simulink model "Trim_Model"  (R2012b)
settings: Solver=ode23tb  StartTime=0.0  StopTime=inf  FixedStep=0.001  MaxStep=0.01  RelTol=1e-5
values from neighbouring files (symbols this model uses):
  a = 2.1117    [SetupComplete.m]
  A_x = 0.015    [SetupComplete.m]
  A_y = A_x    (= 0.015)    [SetupComplete.m]
  A_z = 0.16    [SetupComplete.m]
  C_d0 = 0.00209    [SetupComplete.m]
  C_x = 1.2    [SetupComplete.m]
  C_y = C_x    (= 1.2)    [SetupComplete.m]
  C_z = 2.2    [SetupComplete.m]
  CG_0 = [0,0,0.02]'    [SetupComplete.m]
  h = 0.08    [SetupComplete.m]
  h_FA = 0.02    [SetupComplete.m]
  h_M = 0.064    [SetupComplete.m]
  I_BAC_0 = [ Ix,0,Ixz;0,Iy,0;Ixz,0,Iz]    [SetupComplete.m]
  I_prop = 1/4*M_eq*R^2*diag([1,1,2])    [SetupComplete.m]
  I_tube = [1/2*M_tube*R_tube_eq^2,0,  0  ;           0 ,1/3*M_tube*l_arm^2,0;             0  ,0,1/3*M_tube*l_arm^2]    [SetupComplete.m]
  Initial_Omegas = [1;1;1]*Omega_hover    [Run3Copter.m]
  Initial_Torques = [1;1;1]*Torque_hover    [Run3Copter.m]
  J_FA = I_prop(1,1) + m_prop*h^2  + m_FA*h_FA^2 + m_M*h_M^2    [SetupComplete.m]
  J_T = J_m+1/2*M_eq*R^2    (= 2.000642e-05)    [SetupComplete.m]
  l = 0.345    [SetupComplete.m]
  l_arm = 0.264    [SetupComplete.m]
  m = 3.51    [SetupComplete.m]
  m_0 = 2.61    [SetupComplete.m]
  m_FA = 0.02    [SetupComplete.m]
  m_M = 0.300    (= 0.3)    [SetupComplete.m]
  m_prop = 0.02    [SetupComplete.m]
  Omega_hover = 570    [SetupComplete.m]
  R = 0.1778    [SetupComplete.m]
  rho = 1.15    [SetupComplete.m]
  Rotation_sign = [ 1,-1,-1]    [SetupComplete.m]
  sigma = b*c/(pi*R)    (= 0.107416159567)    [SetupComplete.m]
  Tau_motors = 0.06    [SetupComplete.m]
  theta_0 = 0.38397    [SetupComplete.m]
  theta_1 = -0.2967    [SetupComplete.m]
  Throttle_Hover = X(1)/16    [SetupComplete.m]
  v_i0 = sqrt( 1/3*m*g/(2*rho*pi*R^2)  )    [SetupComplete.m]
undefined symbols (not defined in the file or in its folder): Omega_TTO, Throtle_TTO, Torque_TTO, v_i_adim, Vx_adim, Vz_adim
libraries: vrlib x15, dspmtrx3 x11, simulink_extras x4, aerolibtransform2 x1
(part 1 of 2)
settings Model: ExtModeTrigDuration=5000  Creator=DavidTorres  LastModifiedBy=David
settings SolverCC: SolverResetMethod=Robust  PositivePriorityOrder=on
settings DataIOCC: ExternalInput=getinputstruct(op_trim1)  InitialState=getstatestruct(op_trim1)  SignalLoggingSaveFormat=ModelDataLogs  Refine=10
settings OptimizationCC: InlineParams=on
settings DebuggingCC: FcnCallInpInsideContextMsg=UseLocalSettings
settings RTWCC: SystemTargetFile=quarc_windows.tlc  TemplateMakefile=quarc_default_tmf  Description=QUARC Win32 Target  ProcessScript=quarc_windows_make_rtw_hook
settings STFCustomTargetCC: TargetPreCompLibLocation=C:\PROGRA~2\QUARC\lib\2011a\windows\release  CodeReplacementLibrary=ANSI_C  GeneratePreprocessorConditionals=Disable all  SystemTargetFile=quarc_windows.tlc
settings GRTTargetCC: TargetPreCompLibLocation=C:\PROGRA~2\QUARC\lib\2011a\windows\release  ParMdlRefBuildCompliant=off  CompOptLevelCompliant=off  ConcurrentExecutionCompliant=off  CombineOutputUpdateFcns=off  MatFileLogging=off  GRTInterface=on  ExtMode=on  ExtModeMexFile=quarc_comm

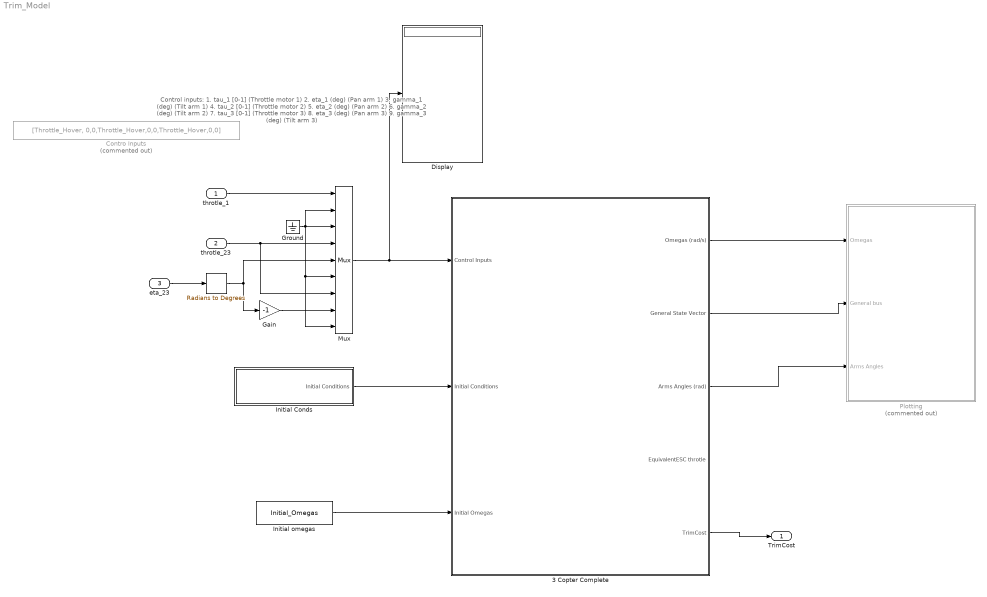
== system Trim_Model ==
  note: Control inputs:
      | 1. tau_1 [0-1] (Throttle motor 1)
      | 2. eta_1 (deg)  (Pan arm 1)
      | 3. gamma_1 (deg)  (Tilt arm 1)
      |
      | 4. tau_2 [0-1] (Throttle motor 2)
      | 5. eta_2 (deg)  (Pan arm 2)
      | 6. gamma_2 (deg)  (Tilt arm 2)
      |
      | 7. tau_3 [0-1] (Throttle motor 3)
      | 8. eta_3 (deg)  (Pan arm  3)
      | 9. gamma_3 (deg)  (Tilt arm 3)
  throtle_1 : Inport
  throtle_23 : Inport  Port=2
  eta_23 : Inport  Port=3
  " " : simulink_extras/Transformations/Radians to Degrees
  3 Copter Complete : Subsystem  TreatAsAtomicUnit=on
  Contro Inputs : Constant  Commented=on  Value=[Throttle_Hover, 0,0,Throttle_Hover,0,0,Throttle_Hover,0,0]
  Display : Display
  Gain : Gain  Gain=-1
  Ground : Ground
  Initial Conds : Subsystem  TreatAsAtomicUnit=on
  Initial omegas : Constant  Value=Initial_Omegas
  Mux : Mux  Inputs=9
  Plotting : Subsystem  Commented=on
  TrimCost : Outport
  wires:
  Initial omegas/1 -> 3 Copter Complete/3(Initial Omegas)
  Initial Conds/1(Initial Conditions) -> 3 Copter Complete/2(Initial Conditions)
  Mux/1 -> Display/1, 3 Copter Complete/1(Control Inputs)
  3 Copter Complete/2(General State Vector) -> Plotting/2(General bus)
  3 Copter Complete/1(Omegas (rad/s)) -> Plotting/1(Omegas)
  3 Copter Complete/3(Arms Angles (rad)) -> Plotting/3(Arms Angles)
  3 Copter Complete/5(TrimCost) -> TrimCost/1
  throtle_1/1 -> Mux/1
  throtle_23/1 -> Mux/7, Mux/4
  Ground/1 -> Mux/2, Mux/6, Mux/9, Mux/3
  eta_23/1 -> " "/1
  " "/1 -> Gain/1, Mux/5
  Gain/1 -> Mux/8

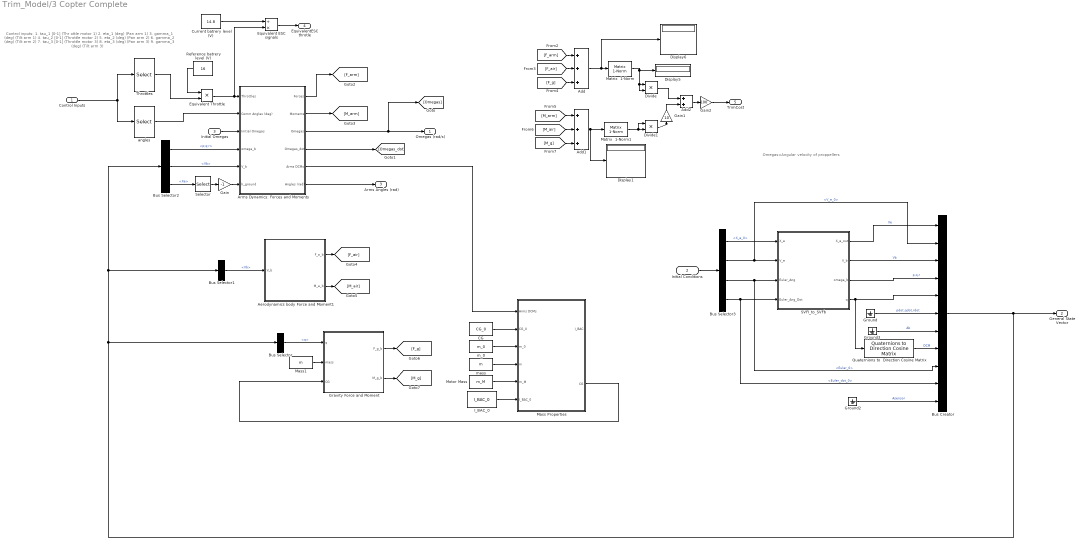
== system Trim_Model/3 Copter Complete ==
  note: Omegas=Angular velocity of proppellers
  note: Control inputs:
      | 1. tau_1 [0-1] (Thr ottle motor 1)
      | 2. eta_1 (deg)  (Pan arm 1)
      | 3. gamma_1 (deg)  (Tilt arm 1)
      |
      | 4. tau_2 [0-1] (Throttle motor 2)
      | 5. eta_2 (deg)  (Pan arm 2)
      | 6. gamma_2 (deg)  (Tilt arm 2)
      |
      | 7. tau_3 [0-1] (Throttle motor 3)
      | 8. eta_3 (deg)  (Pan arm  3)
      | 9. gamma_3 (deg)  (Tilt arm 3)
  Control Inputs : Inport
  Initial Conditions : Inport  Port=2
  Initial Omegas : Inport  Port=3
  Add : Sum  Inputs=+++
  Add1 : Sum  Inputs=+++
  Add2 : Sum
  Aerodynamics body Force and Moment1 : MATLAB Function  TreatAsAtomicUnit=on
  Arms Dynamics: Forces and Moments : Subsystem  TreatAsAtomicUnit=on
  Bus Creator : BusCreator  Inputs=11
  Bus Selector : BusSelector  OutputSignals=q
  Bus Selector1 : BusSelector  OutputSignals=Vb
  Bus Selector2 : BusSelector  OutputSignals=p;q;r,Vb,Xe
  Bus Selector3 : BusSelector  OutputSignals=X_e_0,V_e_0,Euler_0,Euler_dot_0
  CG : Constant  Value=CG_0
  Current batrery level (V) : Constant  Value=14.8
  Display1 : Display
  Display5 : Display
  Display6 : Display
  Divide : Product  Inputs=**
  Divide1 : Product  Inputs=**
  Equivalent ESC signals : Product  Inputs=/*
  Equivalent Throttle : Product  Inputs=**
  Gain : Gain  Gain=-1
  Gain1 : Gain  Gain=10
  Gain2 : Gain  Gain=100
  Gravity Force and Moment : MATLAB Function  TreatAsAtomicUnit=on
  Ground : Ground
  Ground2 : Ground
  Ground3 : Ground
  I_BAC_0 : Constant  Value=I_BAC_0
  Mass Properties : Subsystem  TreatAsAtomicUnit=on
  Mass1 : Constant  Value=m
  Matrix  1-Norm : dspmtrx3/Matrix  1-Norm  outputDataTypeStr=Inherit: Same as accumulator  outputLastDataTypeStr=Inherit: Same as accumulator  outputMin=[]  outputMax=[]  roundingMode=Floor  overflowMode=off
  Matrix  1-Norm1 : dspmtrx3/Matrix  1-Norm  outputDataTypeStr=Inherit: Same as accumulator  outputLastDataTypeStr=Inherit: Same as accumulator  outputMin=[]  outputMax=[]  roundingMode=Floor  overflowMode=off
  Motor Mass : Constant  Value=m_M
  Quaternions to  Direction Cosine Matrix : aerolibtransform2/Quaternions to  Direction Cosine Matrix
  Reference batrery level (V) : Constant  Value=16
  SVFI_to_SVFb : MATLAB Function  TreatAsAtomicUnit=on
  Selector : Selector  InputPortWidth=3  IndexOptions=Index vector (dialog)  Indices=3  OutputSizes=1
  Throttles : Selector  InputPortWidth=9  IndexOptions=Index vector (dialog)  Indices=[1,4,7]  OutputSizes=1
  "angles " : Selector  InputPortWidth=9  IndexOptions=Index vector (dialog)  Indices=[2,3,5,6,8,9]  OutputSizes=1
  m_0 : Constant  Value=m_0
  mass : Constant  Value=m
  Omegas (rad/s) : Outport
  General State Vector : Outport  Port=2
  Arms Angles (rad) : Outport  Port=3
  EquivalentESC throtle : Outport  Port=4
  TrimCost : Outport  Port=5
  wires:
  SVFI_to_SVFb/3(omega_b) -> Bus Creator/4  "p,q,r"
  SVFI_to_SVFb/2(V_b) -> Bus Creator/3  "Vb"
  SVFI_to_SVFb/4(q) -> Quaternions to  Direction Cosine Matrix/1, Bus Creator/5
  Ground/1 -> Bus Creator/6  "pdot,qdot,rdot"
  SVFI_to_SVFb/1(X_e_out) -> Bus Creator/1  "Xe"
  Ground3/1 -> Bus Creator/7  "Ab"
  Bus Selector/1 -> Gravity Force and Moment/1(q)  "<q>"
  Bus Selector1/1 -> Aerodynamics body Force and Moment1/1(V_b)  "<Vb>"
  Bus Selector2/1 -> Arms Dynamics: Forces and Moments/4(omega_b)  "<p;q;r>"
  Bus Selector2/2 -> Arms Dynamics: Forces and Moments/5(V_b)  "<Vb>"
  Mass1/1 -> Gravity Force and Moment/2(mass)
  Mass Properties/2(CG) -> Gravity Force and Moment/3(CG)
  Arms Dynamics: Forces and Moments/4(Omegas_dot) -> [Omegas_dot]
  Initial Omegas/1 -> Arms Dynamics: Forces and Moments/3(Initial Omegas)
  Bus Selector2/3 -> Selector/1  "<Xe>"
  Selector/1 -> Gain/1
  Gain/1 -> Arms Dynamics: Forces and Moments/6(h_ground)
  Arms Dynamics: Forces and Moments/1(Forces) -> [F_arm]
  Arms Dynamics: Forces and Moments/2(Moments) -> [M_arm]
  Aerodynamics body Force and Moment1/1(F_a_b) -> [F_air]
  Aerodynamics body Force and Moment1/2(M_a_b) -> [M_air]
  Gravity Force and Moment/1(F_g_b) -> [F_g]
  Gravity Force and Moment/2(M_g_b) -> [M_g]
  [F_arm] -> Add/1
  [F_air] -> Add/2
  [F_g] -> Add/3
  [M_arm] -> Add1/1
  [M_g] -> Add1/3
  [M_air] -> Add1/2
  Ground2/1 -> Bus Creator/11  "Asensor"
  Throttles/1 -> Equivalent Throttle/2
  Control Inputs/1 -> "angles "/1, Throttles/1
  "angles "/1 -> Arms Dynamics: Forces and Moments/2(Comm Angles (deg))
  Arms Dynamics: Forces and Moments/5(Arms DCMs) -> Mass Properties/1(Arms DCMs)
  CG/1 -> Mass Properties/2(CG_0)
  Motor Mass/1 -> Mass Properties/5(m_M)
  I_BAC_0/1 -> Mass Properties/6(I_BAC_0)
  m_0/1 -> Mass Properties/3(m_0)
  mass/1 -> Mass Properties/4(m)
  Arms Dynamics: Forces and Moments/3(Omegas) -> [Omegas], Omegas (rad/s)/1
  Arms Dynamics: Forces and Moments/6(Angles (rad)) -> Arms Angles (rad)/1
  Bus Creator/1 -> Bus Selector2/1, Bus Selector1/1, Bus Selector/1, General State Vector/1
  Equivalent Throttle/1 -> Equivalent ESC signals/2, Arms Dynamics: Forces and Moments/1(Throttles)
  Reference batrery level (V)/1 -> Equivalent Throttle/1
  Current batrery level (V)/1 -> Equivalent ESC signals/1
  Equivalent ESC signals/1 -> EquivalentESC throtle/1
  Initial Conditions/1 -> Bus Selector3/1
  Bus Selector3/1 -> SVFI_to_SVFb/1(X_e)  "<X_e_0>"
  Bus Selector3/2 -> Bus Creator/2, SVFI_to_SVFb/2(V_e)  "<V_e_0>"
  Bus Selector3/3 -> Bus Creator/9, SVFI_to_SVFb/3(Euler_Ang)  "<Euler_0>"
  Bus Selector3/4 -> Bus Creator/10, SVFI_to_SVFb/4(Euler_Ang_Dot)  "<Euler_dot_0>"
  Quaternions to  Direction Cosine Matrix/1 -> Bus Creator/8  "DCM"
  Add/1 -> Display6/1, Matrix  1-Norm/1
  Add1/1 -> Display1/1, Matrix  1-Norm1/1
  Add2/1 -> Gain2/1
  Gain1/1 -> Add2/2
  Matrix  1-Norm1/1 -> Divide1/1, Divide1/2
  Matrix  1-Norm/1 -> Divide/2, Divide/1, Display5/1
  Gain2/1 -> TrimCost/1
  Divide/1 -> Add2/1
  Divide1/1 -> Gain1/1

== system Trim_Model/Initial Conds ==
  Bus Creator : BusCreator
  Ini Position X_e_0 : Constant  Value=[0;0;-20]
  Initial Attitude Euler_0 : Constant  Value=[deg2rad(0);deg2rad(0);deg2rad(0)]
  Initial Attitude Rate  Euler_dot_0 : Constant  Value=[deg2rad(0);deg2rad(0);deg2rad(0)]
  Initial Velocity V_e_0 : Constant  Value=[0;0;0]
  Initial Conditions : Outport
  wires:
  Ini Position X_e_0/1 -> Bus Creator/1  "X_e_0"
  Initial Velocity V_e_0/1 -> Bus Creator/2  "V_e_0"
  Initial Attitude Euler_0/1 -> Bus Creator/3  "Euler_0"
  Initial Attitude Rate  Euler_dot_0/1 -> Bus Creator/4  "Euler_dot_0"
  Bus Creator/1 -> Initial Conditions/1

== system Trim_Model/Plotting ==
  Omegas : Inport
  General bus : Inport  Port=2
  Arms Angles : Inport  Port=3
  Bus Selector : BusSelector  OutputSignals=euler,Xe
  Bus Selector1 : BusSelector  OutputSignals=Angles Arm 1,Angles Arm 2,Angles Arm 3
  Scope : Scope  NumInputPorts=2
      settings: YMin=-3.5~-110  YMax=3.5~40
  Scope1 : Scope
      settings: TimeRange=5  YMin=0  YMax=700
  Scope2 : Scope  NumInputPorts=3
      settings: ShowLegends=on  YMin=-5~-5~-5  YMax=5~5~5  SaveName=ScopeData2
  wires:
  General bus/1 -> Bus Selector/1
  Bus Selector/1 -> Scope/1  "<euler>"
  Omegas/1 -> Scope1/1  "Omegas"
  Arms Angles/1 -> Bus Selector1/1
  Bus Selector1/3 -> Scope2/3  "<Angles Arm 3>"
  Bus Selector1/2 -> Scope2/2  "<Angles Arm 2>"
  Bus Selector1/1 -> Scope2/1  "<Angles Arm 1>"
  Bus Selector/2 -> Scope/2  "<Xe>"

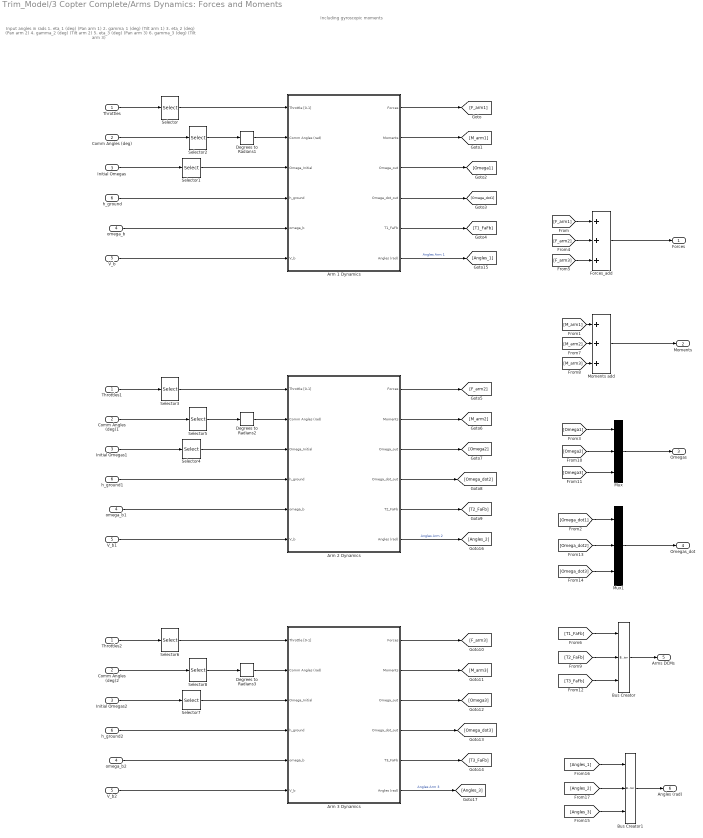
== system Trim_Model/3 Copter Complete/Arms Dynamics: Forces and Moments ==
  note: Including gyroscopic moments
  note: Input angles in rads
      |
      | 1. eta_1 (deg)  (Pan arm 1)
      | 2. gamma_1 (deg)  (Tilt arm 1)
      |
      | 3. eta_2 (deg)  (Pan arm 2)
      | 4. gamma_2 (deg)  (Tilt arm 2)
      |
      | 5. eta_3 (deg)  (Pan arm  3)
      | 6. gamma_3 (deg)  (Tilt arm 3)
  Throttles : Inport
  Comm Angles (deg) : Inport  Port=2
  Initial Omegas : Inport  Port=3
  omega_b : Inport  Port=4
  V_b : Inport  Port=5
  h_ground : Inport  Port=6
  Arm 1 Dynamics : Subsystem  TreatAsAtomicUnit=on
  Arm 2 Dynamics : Subsystem  TreatAsAtomicUnit=on
  Arm 3 Dynamics : Subsystem  TreatAsAtomicUnit=on
  Bus Creator : BusCreator  Inputs=3
  Bus Creator1 : BusCreator  Inputs=3
  Comm Angles (deg)1 : InportShadow  Port=2
  Comm Angles (deg)2 : InportShadow  Port=2
  Degrees to Radians1 : simulink_extras/Transformations/Degrees to Radians
  Degrees to Radians2 : simulink_extras/Transformations/Degrees to Radians
  Degrees to Radians3 : simulink_extras/Transformations/Degrees to Radians
  Forces_add : Sum  Inputs=+++
  Initial Omegas1 : InportShadow  Port=3
  Initial Omegas2 : InportShadow  Port=3
  Moments add : Sum  Inputs=+++
  Mux : Mux  Inputs=3
  Mux1 : Mux  Inputs=3
  Selector : Selector  InputPortWidth=3  IndexOptions=Index vector (dialog)  Indices=[1]  OutputSizes=1
  Selector1 : Selector  InputPortWidth=3  IndexOptions=Index vector (dialog)  Indices=[1]  OutputSizes=1
  Selector2 : Selector  InputPortWidth=6  IndexOptions=Index vector (dialog)  Indices=[1,2]  OutputSizes=1
  Selector3 : Selector  InputPortWidth=3  IndexOptions=Index vector (dialog)  Indices=2  OutputSizes=1
  Selector4 : Selector  InputPortWidth=3  IndexOptions=Index vector (dialog)  Indices=2  OutputSizes=1
  Selector5 : Selector  InputPortWidth=6  IndexOptions=Index vector (dialog)  Indices=[3,4]  OutputSizes=1
  Selector6 : Selector  InputPortWidth=3  IndexOptions=Index vector (dialog)  Indices=3  OutputSizes=1
  Selector7 : Selector  InputPortWidth=3  IndexOptions=Index vector (dialog)  Indices=3  OutputSizes=1
  Selector8 : Selector  InputPortWidth=6  IndexOptions=Index vector (dialog)  Indices=[5,6]  OutputSizes=1
  Throttles1 : InportShadow
  Throttles2 : InportShadow
  V_b1 : InportShadow  Port=5
  V_b2 : InportShadow  Port=5
  h_ground1 : InportShadow  Port=6
  h_ground2 : InportShadow  Port=6
  omega_b1 : InportShadow  Port=4
  omega_b2 : InportShadow  Port=4
  Forces : Outport
  Moments : Outport  Port=2
  Omegas : Outport  Port=3
  Omegas_dot : Outport  Port=4
  Arms DCMs : Outport  Port=5
  Angles (rad) : Outport  Port=6
  wires:
  Selector1/1 -> Arm 1 Dynamics/3(Omega_Initial)
  Throttles/1 -> Selector/1
  Initial Omegas/1 -> Selector1/1
  Selector/1 -> Arm 1 Dynamics/1(Throttle [0-1])
  V_b/1 -> Arm 1 Dynamics/6(V_b)
  Forces_add/1 -> Forces/1
  Moments add/1 -> Moments/1
  Mux/1 -> Omegas/1
  Mux1/1 -> Omegas_dot/1
  h_ground/1 -> Arm 1 Dynamics/4(h_ground)
  Arm 1 Dynamics/1(Forces) -> [F_arm1]
  Arm 1 Dynamics/2(Moments) -> [M_arm1]
  Arm 1 Dynamics/3(Omega_out) -> [Omega1]
  Arm 1 Dynamics/4(Omega_dot_out) -> [Omega_dot1]
  [F_arm1] -> Forces_add/1
  [M_arm1] -> Moments add/1
  [Omega_dot1] -> Mux1/1
  [Omega1] -> Mux/1
  omega_b/1 -> Arm 1 Dynamics/5(omega_b)
  [F_arm2] -> Forces_add/2
  [F_arm3] -> Forces_add/3
  [Omega2] -> Mux/2
  [Omega3] -> Mux/3
  [Omega_dot2] -> Mux1/2
  [Omega_dot3] -> Mux1/3
  [M_arm3] -> Moments add/3
  [M_arm2] -> Moments add/2
  Degrees to Radians1/1 -> Arm 1 Dynamics/2(Comm Angles (rad))
  Comm Angles (deg)/1 -> Selector2/1
  Selector2/1 -> Degrees to Radians1/1
  Arm 1 Dynamics/5(T1_FaFb) -> [T1_FaFb]
  Bus Creator/1 -> Arms DCMs/1
  [T1_FaFb] -> Bus Creator/1
  Selector4/1 -> Arm 2 Dynamics/3(Omega_Initial)
  Throttles1/1 -> Selector3/1
  Initial Omegas1/1 -> Selector4/1
  Selector3/1 -> Arm 2 Dynamics/1(Throttle [0-1])
  V_b1/1 -> Arm 2 Dynamics/6(V_b)
  h_ground1/1 -> Arm 2 Dynamics/4(h_ground)
  Arm 2 Dynamics/1(Forces) -> [F_arm2]
  Arm 2 Dynamics/2(Moments) -> [M_arm2]
  Arm 2 Dynamics/3(Omega_out) -> [Omega2]
  Arm 2 Dynamics/4(Omega_dot_out) -> [Omega_dot2]
  omega_b1/1 -> Arm 2 Dynamics/5(omega_b)
  Degrees to Radians2/1 -> Arm 2 Dynamics/2(Comm Angles (rad))
  Comm Angles (deg)1/1 -> Selector5/1
  Selector5/1 -> Degrees to Radians2/1
  Arm 2 Dynamics/5(T2_FaFb) -> [T2_FaFb]
  [T2_FaFb] -> Bus Creator/2
  Selector7/1 -> Arm 3 Dynamics/3(Omega_Initial)
  Throttles2/1 -> Selector6/1
  Initial Omegas2/1 -> Selector7/1
  Selector6/1 -> Arm 3 Dynamics/1(Throttle [0-1])
  V_b2/1 -> Arm 3 Dynamics/6(V_b)
  h_ground2/1 -> Arm 3 Dynamics/4(h_ground)
  Arm 3 Dynamics/1(Forces) -> [F_arm3]
  Arm 3 Dynamics/2(Moments) -> [M_arm3]
  Arm 3 Dynamics/3(Omega_out) -> [Omega3]
  Arm 3 Dynamics/4(Omega_dot_out) -> [Omega_dot3]
  omega_b2/1 -> Arm 3 Dynamics/5(omega_b)
  Degrees to Radians3/1 -> Arm 3 Dynamics/2(Comm Angles (rad))
  Comm Angles (deg)2/1 -> Selector8/1
  Selector8/1 -> Degrees to Radians3/1
  Arm 3 Dynamics/5(T3_FaFb) -> [T3_FaFb]
  [T3_FaFb] -> Bus Creator/3
  Bus Creator1/1 -> Angles (rad)/1
  [Angles_1] -> Bus Creator1/1
  [Angles_2] -> Bus Creator1/2
  [Angles_3] -> Bus Creator1/3
  Arm 1 Dynamics/6(Angles (rad)) -> [Angles_1]  "Angles Arm 1"
  Arm 2 Dynamics/6(Angles (rad)) -> [Angles_2]  "Angles Arm 2"
  Arm 3 Dynamics/6(Angles (rad)) -> [Angles_3]  "Angles Arm 3"

== system Trim_Model/3 Copter Complete/Mass Properties ==
  Arms DCMs : Inport
  CG_0 : Inport  Port=2
  m_0 : Inport  Port=3
  m : Inport  Port=4
  m_M : Inport  Port=5
  I_BAC_0 : Inport  Port=6
  Arm Inertia : MATLAB Function  TreatAsAtomicUnit=on
  Bus Selector : BusSelector  OutputSignals=T^1_F_a;Fb,T^2_F_a;Fb,T^3_F_a;Fb
  CG position : Sum
  Divide : Product  Inputs=*/
  Divide1 : Product  Inputs=**
  Divide2 : Product  Inputs=/*
  Divide3 : Product  Inputs=**
  Motors Pos sum : Sum  Inputs=+++
  Total I_BAC : Sum
  I_BAC : Outport
  CG : Outport  Port=2
  wires:
  Arms DCMs/1 -> Bus Selector/1
  Bus Selector/3 -> Arm Inertia/3(T3_FAFb)  "<T^3_F_a;Fb>"
  Bus Selector/2 -> Arm Inertia/2(T2_FAFb)  "<T^2_F_a;Fb>"
  Bus Selector/1 -> Arm Inertia/1(T1_FAFb)  "<T^1_F_a;Fb>"
  Total I_BAC/1 -> I_BAC/1
  m_0/1 -> Divide/1
  m/1 -> Divide/2, Divide2/1
  CG_0/1 -> Divide1/1
  Divide/1 -> Divide1/2
  m_M/1 -> Divide2/2
  CG position/1 -> CG/1
  Divide1/1 -> CG position/1
  Motors Pos sum/1 -> Divide3/1
  Divide2/1 -> Divide3/2
  Divide3/1 -> CG position/2
  Arm Inertia/3(r2_M) -> Motors Pos sum/2
  Arm Inertia/4(r3_M) -> Motors Pos sum/1
  Arm Inertia/1(I_M) -> Total I_BAC/2
  I_BAC_0/1 -> Total I_BAC/1
  Arm Inertia/2(r1_M) -> Motors Pos sum/3

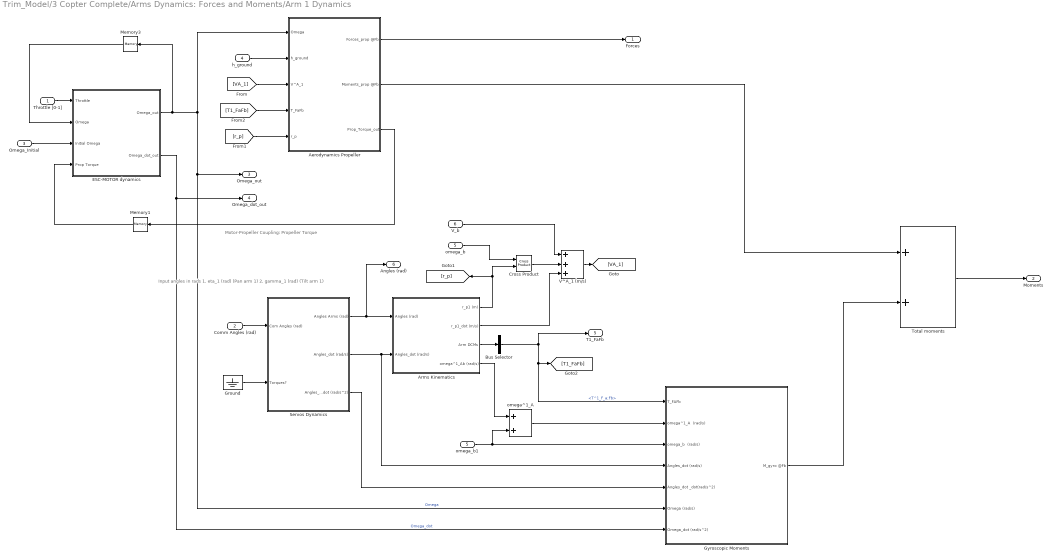
== system Trim_Model/3 Copter Complete/Arms Dynamics: Forces and Moments/Arm 1 Dynamics ==
  note: Motor-Propeller Coupling: Propeller Torque
  note: Input angles in rads
      |
      | 1. eta_1 (rad)  (Pan arm 1)
      | 2. gamma_1 (rad)  (Tilt arm 1)
  Throttle [0-1] : Inport
  Comm Angles (rad) : Inport  Port=2
  Omega_Initial : Inport  Port=3
  h_ground : Inport  Port=4
  omega_b : Inport  Port=5
  V_b : Inport  Port=6
  Aerodynamics Propeller : Subsystem  TreatAsAtomicUnit=on
      settings: MinAlgLoopOccurrences=on
  Arms Kinematics : Subsystem  TreatAsAtomicUnit=on
  Bus Selector : BusSelector  OutputSignals=T^1_F_a;Fb
  Cross Product : vrlib/Utilities/Cross Product
  ESC-MOTOR dynamics : Subsystem  Variant=on  OverrideUsingVariant=Variant_completed
  Ground : Ground
  Gyroscopic Moments : Subsystem  TreatAsAtomicUnit=on
  Memory1 : Memory  X0=Initial_Torques(1)
  Memory3 : Memory  X0=Initial_Omegas(1)
  Servos Dynamics : Subsystem  TreatAsAtomicUnit=on
  Total moments : Sum
  V^A_1 (m/s) : Sum  Inputs=+++
  omega^1_A : Sum
  omega_b1 : InportShadow  Port=5
  Forces : Outport
  Moments : Outport  Port=2
  Omega_out : Outport  Port=3
  Omega_dot_out : Outport  Port=4
  T1_FaFb : Outport  Port=5
  Angles (rad) : Outport  Port=6
  wires:
  Throttle [0-1]/1 -> ESC-MOTOR dynamics/1(Throttle)
  Omega_Initial/1 -> ESC-MOTOR dynamics/3(Initial Omega)
  ESC-MOTOR dynamics/2(Omega_dot_out) -> Gyroscopic Moments/7(Omega_dot (rad/s^2)), Omega_dot_out/1  "Omega_dot"
  ESC-MOTOR dynamics/1(Omega_out) -> Memory3/1, Omega_out/1, Gyroscopic Moments/6(Omega (rad/s)), Aerodynamics Propeller/1(Omega)  "Omega"
  h_ground/1 -> Aerodynamics Propeller/2(h_ground)
  Comm Angles (rad)/1 -> Servos Dynamics/1(Com Angles (rad))
  Servos Dynamics/1(Angles Arms (rad)) -> Angles (rad)/1, Arms Kinematics/1(Angles (rad))
  omega_b/1 -> Cross Product/1
  Arms Kinematics/1(r_p1 (m)) -> [r_p], Cross Product/2
  Cross Product/1 -> V^A_1 (m/s)/2
  V_b/1 -> V^A_1 (m/s)/1
  Arms Kinematics/2(r_p1_dot (m/s)) -> V^A_1 (m/s)/3
  V^A_1 (m/s)/1 -> [VA_1]
  [VA_1] -> Aerodynamics Propeller/3(V^A_1)
  [T1_FaFb] -> Aerodynamics Propeller/4(T_FaFb)
  Arms Kinematics/3(Arm DCMs) -> Bus Selector/1
  Bus Selector/1 -> T1_FaFb/1, Gyroscopic Moments/1(T_FAFb), [T1_FaFb]  "<T^1_F_a;Fb>"
  [r_p] -> Aerodynamics Propeller/5(r_p)
  Aerodynamics Propeller/1(Forces_prop @Fb) -> Forces/1
  Servos Dynamics/2(Angles_dot (rad/s)) -> Gyroscopic Moments/4(Angles_dot (rad/s)), Arms Kinematics/2(Angles_dot (rad/s))
  Arms Kinematics/4(omega^1_Ab (rad/s)) -> omega^1_A/1
  omega_b1/1 -> Gyroscopic Moments/3(omega_b  (rad/s)), omega^1_A/2
  omega^1_A/1 -> Gyroscopic Moments/2(omega^1_A  (rad/s))
  Servos Dynamics/3(Angles_dot_dot (rad/s^2)) -> Gyroscopic Moments/5(Angles_dot _dot(rad/s^2))
  Ground/1 -> Servos Dynamics/2(Torques?)
  Aerodynamics Propeller/2(Moments_prop @Fb) -> Total moments/1
  Gyroscopic Moments/1(M_gyro @Fb) -> Total moments/2
  Total moments/1 -> Moments/1
  Aerodynamics Propeller/3(Prop_Torque_out) -> Memory1/1
  Memory1/1 -> ESC-MOTOR dynamics/4(Prop Torque)
  Memory3/1 -> ESC-MOTOR dynamics/2(Omega)

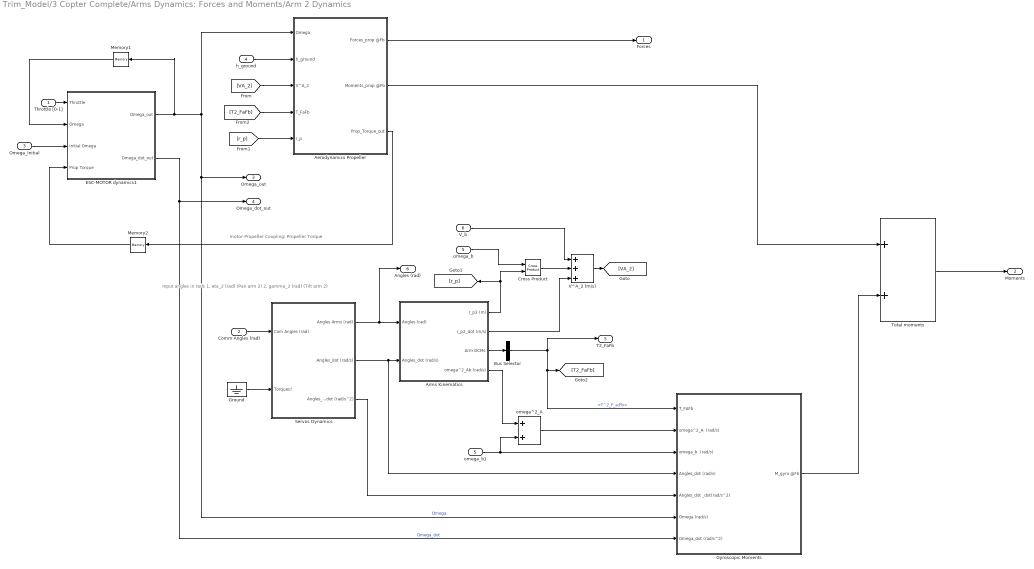
== system Trim_Model/3 Copter Complete/Arms Dynamics: Forces and Moments/Arm 2 Dynamics ==
  note: Input angles in rads
      |
      | 1. eta_2 (rad)  (Pan arm 2)
      | 2. gamma_2 (rad)  (Tilt arm 2)
  note: motor-Propeller Coupling: Propeller Torque
  Throttle [0-1] : Inport
  Comm Angles (rad) : Inport  Port=2
  Omega_Initial : Inport  Port=3
  h_ground : Inport  Port=4
  omega_b : Inport  Port=5
  V_b : Inport  Port=6
  Aerodynamics Propeller : Subsystem  TreatAsAtomicUnit=on
  Arms Kinematics : Subsystem  TreatAsAtomicUnit=on
  Bus Selector : BusSelector  OutputSignals=T^2_F_a;Fb
  Cross Product : vrlib/Utilities/Cross Product
  ESC-MOTOR dynamics1 : Subsystem  Variant=on  OverrideUsingVariant=Variant_completed
  Ground : Ground
  Gyroscopic Moments : Subsystem  TreatAsAtomicUnit=on
  Memory1 : Memory  X0=Initial_Omegas(2)
  Memory2 : Memory  X0=Initial_Torques(2)
  Servos Dynamics : Subsystem  TreatAsAtomicUnit=on
  Total moments : Sum
  V^A_2 (m/s) : Sum  Inputs=+++
  omega^2_A : Sum
  omega_b1 : InportShadow  Port=5
  Forces : Outport
  Moments : Outport  Port=2
  Omega_out : Outport  Port=3
  Omega_dot_out : Outport  Port=4
  T2_FaFb : Outport  Port=5
  Angles (rad) : Outport  Port=6
  wires:
  Total moments/1 -> Moments/1
  Gyroscopic Moments/1(M_gyro @Fb) -> Total moments/2
  Aerodynamics Propeller/2(Moments_prop @Fb) -> Total moments/1
  Ground/1 -> Servos Dynamics/2(Torques?)
  Servos Dynamics/3(Angles_dot_dot (rad/s^2)) -> Gyroscopic Moments/5(Angles_dot _dot(rad/s^2))
  omega^2_A/1 -> Gyroscopic Moments/2(omega^2_A  (rad/s))
  omega_b1/1 -> omega^2_A/2, Gyroscopic Moments/3(omega_b  (rad/s))
  Arms Kinematics/4(omega^2_Ab (rad/s)) -> omega^2_A/1
  Servos Dynamics/2(Angles_dot (rad/s)) -> Gyroscopic Moments/4(Angles_dot (rad/s)), Arms Kinematics/2(Angles_dot (rad/s))
  Aerodynamics Propeller/1(Forces_prop @Fb) -> Forces/1
  [r_p] -> Aerodynamics Propeller/5(r_p)
  Bus Selector/1 -> [T2_FaFb], Gyroscopic Moments/1(T_FAFb), T2_FaFb/1  "<T^2_F_a;Fb>"
  Arms Kinematics/3(Arm DCMs) -> Bus Selector/1
  [T2_FaFb] -> Aerodynamics Propeller/4(T_FaFb)
  [VA_2] -> Aerodynamics Propeller/3(V^A_2)
  V^A_2 (m/s)/1 -> [VA_2]
  Arms Kinematics/2(r_p2_dot (m/s)) -> V^A_2 (m/s)/3
  V_b/1 -> V^A_2 (m/s)/1
  Cross Product/1 -> V^A_2 (m/s)/2
  Arms Kinematics/1(r_p2 (m)) -> Cross Product/2, [r_p]
  omega_b/1 -> Cross Product/1
  Comm Angles (rad)/1 -> Servos Dynamics/1(Com Angles (rad))
  h_ground/1 -> Aerodynamics Propeller/2(h_ground)
  ESC-MOTOR dynamics1/1(Omega_out) -> Memory1/1, Aerodynamics Propeller/1(Omega), Gyroscopic Moments/6(Omega (rad/s)), Omega_out/1  "Omega"
  ESC-MOTOR dynamics1/2(Omega_dot_out) -> Omega_dot_out/1, Gyroscopic Moments/7(Omega_dot (rad/s^2))  "Omega_dot"
  Omega_Initial/1 -> ESC-MOTOR dynamics1/3(Initial Omega)
  Throttle [0-1]/1 -> ESC-MOTOR dynamics1/1(Throttle)
  Servos Dynamics/1(Angles Arms (rad)) -> Angles (rad)/1, Arms Kinematics/1(Angles (rad))
  Aerodynamics Propeller/3(Prop_Torque_out) -> Memory2/1
  Memory1/1 -> ESC-MOTOR dynamics1/2(Omega)
  Memory2/1 -> ESC-MOTOR dynamics1/4(Prop Torque)

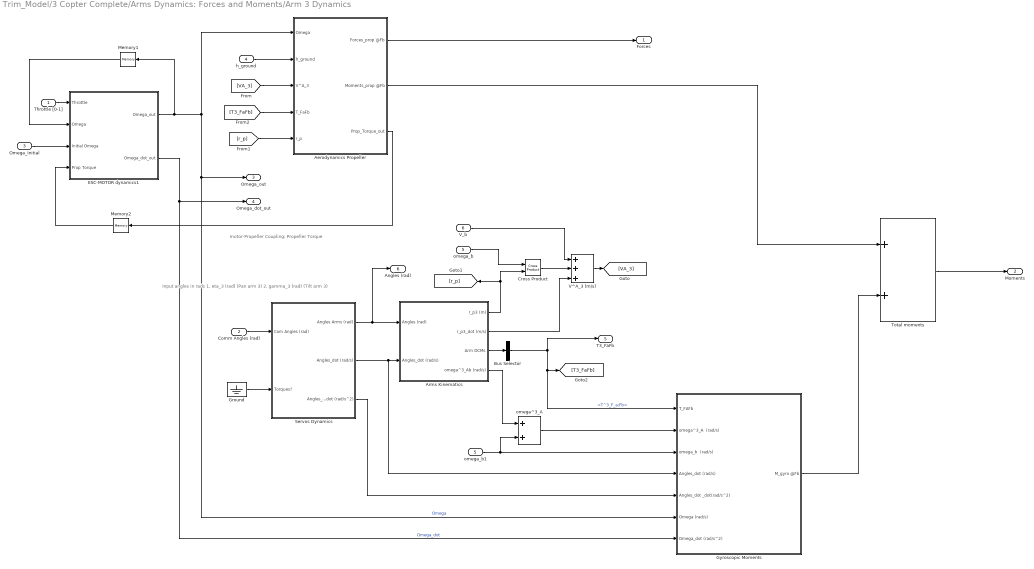
== system Trim_Model/3 Copter Complete/Arms Dynamics: Forces and Moments/Arm 3 Dynamics ==
  note: motor-Propeller Coupling: Propeller Torque
  note: Input angles in rads
      |
      | 1. eta_3 (rad)  (Pan arm 3)
      | 2. gamma_3 (rad)  (Tilt arm 3)
  Throttle [0-1] : Inport
  Comm Angles (rad) : Inport  Port=2
  Omega_Initial : Inport  Port=3
  h_ground : Inport  Port=4
  omega_b : Inport  Port=5
  V_b : Inport  Port=6
  Aerodynamics Propeller : Subsystem  TreatAsAtomicUnit=on
  Arms Kinematics : Subsystem  TreatAsAtomicUnit=on
  Bus Selector : BusSelector  OutputSignals=T^3_F_a;Fb
  Cross Product : vrlib/Utilities/Cross Product
  ESC-MOTOR dynamics1 : Subsystem  Variant=on  OverrideUsingVariant=Variant_completed
  Ground : Ground
  Gyroscopic Moments : Subsystem  TreatAsAtomicUnit=on
  Memory1 : Memory  X0=Initial_Omegas(3)
  Memory2 : Memory  X0=Initial_Torques(3)
  Servos Dynamics : Subsystem  TreatAsAtomicUnit=on
  Total moments : Sum
  V^A_3 (m/s) : Sum  Inputs=+++
  omega^3_A : Sum
  omega_b1 : InportShadow  Port=5
  Forces : Outport
  Moments : Outport  Port=2
  Omega_out : Outport  Port=3
  Omega_dot_out : Outport  Port=4
  T3_FaFb : Outport  Port=5
  Angles (rad) : Outport  Port=6
  wires:
  Throttle [0-1]/1 -> ESC-MOTOR dynamics1/1(Throttle)
  Omega_Initial/1 -> ESC-MOTOR dynamics1/3(Initial Omega)
  ESC-MOTOR dynamics1/2(Omega_dot_out) -> Gyroscopic Moments/7(Omega_dot (rad/s^2)), Omega_dot_out/1  "Omega_dot"
  ESC-MOTOR dynamics1/1(Omega_out) -> Memory1/1, Omega_out/1, Gyroscopic Moments/6(Omega (rad/s)), Aerodynamics Propeller/1(Omega)  "Omega"
  h_ground/1 -> Aerodynamics Propeller/2(h_ground)
  Comm Angles (rad)/1 -> Servos Dynamics/1(Com Angles (rad))
  omega_b/1 -> Cross Product/1
  Arms Kinematics/1(r_p3 (m)) -> [r_p], Cross Product/2
  Cross Product/1 -> V^A_3 (m/s)/2
  V_b/1 -> V^A_3 (m/s)/1
  Arms Kinematics/2(r_p3_dot (m/s)) -> V^A_3 (m/s)/3
  V^A_3 (m/s)/1 -> [VA_3]
  [VA_3] -> Aerodynamics Propeller/3("V^A_3 ")
  [T3_FaFb] -> Aerodynamics Propeller/4(T_FaFb)
  Arms Kinematics/3(Arm DCMs) -> Bus Selector/1
  Bus Selector/1 -> T3_FaFb/1, Gyroscopic Moments/1(T_FAFb), [T3_FaFb]  "<T^3_F_a;Fb>"
  [r_p] -> Aerodynamics Propeller/5(r_p)
  Aerodynamics Propeller/1(Forces_prop @Fb) -> Forces/1
  Servos Dynamics/2(Angles_dot (rad/s)) -> Arms Kinematics/2(Angles_dot (rad/s)), Gyroscopic Moments/4(Angles_dot (rad/s))
  Arms Kinematics/4(omega^3_Ab (rad/s)) -> omega^3_A/1
  omega_b1/1 -> Gyroscopic Moments/3(omega_b  (rad/s)), omega^3_A/2
  omega^3_A/1 -> Gyroscopic Moments/2(omega^3_A  (rad/s))
  Servos Dynamics/3(Angles_dot_dot (rad/s^2)) -> Gyroscopic Moments/5(Angles_dot _dot(rad/s^2))
  Ground/1 -> Servos Dynamics/2(Torques?)
  Aerodynamics Propeller/2(Moments_prop @Fb) -> Total moments/1
  Gyroscopic Moments/1(M_gyro @Fb) -> Total moments/2
  Total moments/1 -> Moments/1
  Servos Dynamics/1(Angles Arms (rad)) -> Angles (rad)/1, Arms Kinematics/1(Angles (rad))
  Aerodynamics Propeller/3(Prop_Torque_out) -> Memory2/1
  Memory1/1 -> ESC-MOTOR dynamics1/2(Omega)
  Memory2/1 -> ESC-MOTOR dynamics1/4(Prop Torque)

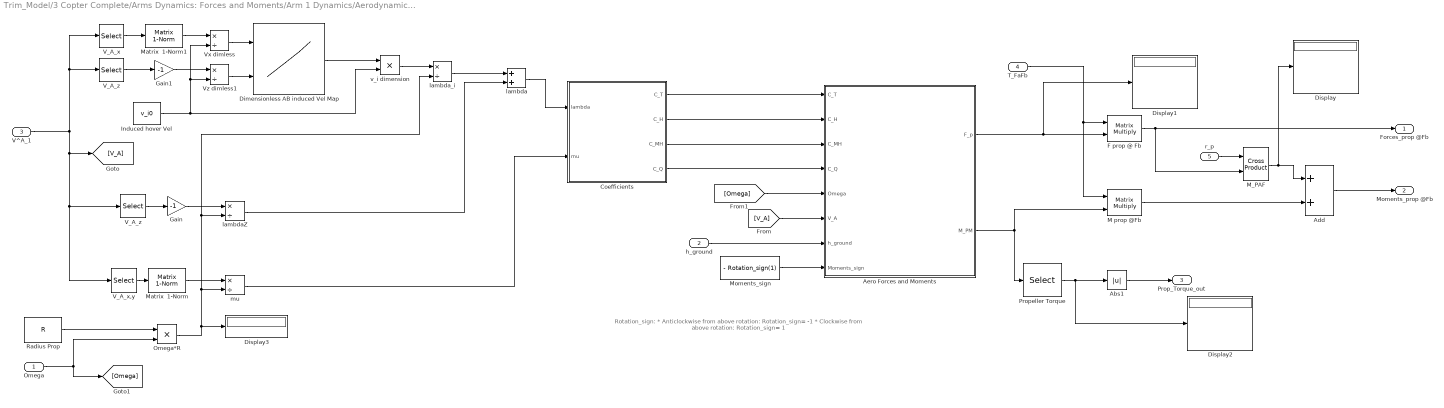
== system Trim_Model/3 Copter Complete/Arms Dynamics: Forces and Moments/Arm 1 Dynamics/Aerodynamics Propeller ==
  note: Rotation_sign:
      |
      | * Anticlockwise from above rotation: Rotation_sign= -1
      | * Clockwise from above rotation: Rotation_sign= 1
  Omega : Inport
  h_ground : Inport  Port=2
  V^A_1 : Inport  Port=3
  T_FaFb : Inport  Port=4
  r_p : Inport  Port=5
  Abs1 : Abs
  Add : Sum
  Aero Forces and Moments : MATLAB Function  TreatAsAtomicUnit=on
  Coefficients : MATLAB Function  TreatAsAtomicUnit=on
  Dimensionless AB induced Vel Map : Lookup_n-D  BreakpointsForDimension1=Vx_adim  BreakpointsForDimension2=Vz_adim  BreakpointsForDimension3=[5, 7]  Table=v_i_adim  ExtrapMethod=Clip  RndMeth=Simplest  InputSameDT=on
  Display{,1..3} (4 alike) : Display
  F prop @ Fb : Product  Multiplication=Matrix(*)
  Gain : Gain  Gain=-1
  Gain1 : Gain  Gain=-1
  Induced hover Vel : Constant  Value=v_i0
  M prop @Fb : Product  Multiplication=Matrix(*)
  M_PAF : vrlib/Utilities/Cross Product
  Matrix  1-Norm : dspmtrx3/Matrix  1-Norm  outputDataTypeStr=Inherit: Same as accumulator  outputLastDataTypeStr=Inherit: Same as accumulator  outputMin=[]  outputMax=[]  roundingMode=Floor  overflowMode=off
  Matrix  1-Norm1 : dspmtrx3/Matrix  1-Norm  outputDataTypeStr=Inherit: Same as accumulator  outputLastDataTypeStr=Inherit: Same as accumulator  outputMin=[]  outputMax=[]  roundingMode=Floor  overflowMode=off
  Moments_sign : Constant  Value=- Rotation_sign(1)
  Omega*R : Product  Inputs=**
  Propeller Torque : Selector  InputPortWidth=3  IndexOptions=Index vector (dialog)  Indices=3  OutputSizes=1
  Radius Prop : Constant  Value=R
  V_A_x : Selector  InputPortWidth=3  IndexOptions=Index vector (dialog)  Indices=[1 2]  OutputSizes=1
  V_A_x,y : Selector  InputPortWidth=3  IndexOptions=Index vector (dialog)  Indices=[1 2]  OutputSizes=1
  V_A_z : Selector  InputPortWidth=3  IndexOptions=Index vector (dialog)  Indices=3  OutputSizes=1
  "V_A_z " : Selector  InputPortWidth=3  IndexOptions=Index vector (dialog)  Indices=[3]  OutputSizes=1
  Vx dimless : Product  Inputs=*/
  Vz dimless1 : Product  Inputs=*/
  lambda : Sum
  lambdaZ : Product  Inputs=*/
  lambda_i : Product  Inputs=*/
  mu : Product  Inputs=*/
  v_i dimension : Product  Inputs=**
  Forces_prop @Fb : Outport
  Moments_prop @Fb : Outport  Port=2
  Prop_Torque_out : Outport  Port=3
  wires:
  Radius Prop/1 -> Omega*R/1
  Omega/1 -> Omega*R/2, [Omega]
  V^A_1/1 -> [V_A], "V_A_z "/1, V_A_x,y/1, V_A_x/1, V_A_z/1
  V_A_x,y/1 -> Matrix  1-Norm/1
  Matrix  1-Norm/1 -> mu/1
  Omega*R/1 -> mu/2, lambdaZ/2, lambda_i/2, Display3/1
  Vx dimless/1 -> Dimensionless AB induced Vel Map/1
  V_A_x/1 -> Matrix  1-Norm1/1
  Vz dimless1/1 -> Dimensionless AB induced Vel Map/2
  V_A_z/1 -> Gain1/1
  Induced hover Vel/1 -> v_i dimension/2, Vz dimless1/2, Vx dimless/2
  Dimensionless AB induced Vel Map/1 -> v_i dimension/1
  v_i dimension/1 -> lambda_i/1
  "V_A_z "/1 -> Gain/1
  Gain/1 -> lambdaZ/1
  lambda_i/1 -> lambda/1
  lambdaZ/1 -> lambda/2
  Gain1/1 -> Vz dimless1/1
  lambda/1 -> Coefficients/1(lambda)
  Coefficients/1(C_T) -> Aero Forces and Moments/1(C_T)
  Coefficients/2(C_H) -> Aero Forces and Moments/2(C_H)
  Coefficients/3(C_MH) -> Aero Forces and Moments/3(C_MH)
  [V_A] -> Aero Forces and Moments/6(V_A)
  [Omega] -> Aero Forces and Moments/5(Omega)
  Aero Forces and Moments/2(M_PM) -> Propeller Torque/1, M prop @Fb/2
  Add/1 -> Moments_prop @Fb/1
  h_ground/1 -> Aero Forces and Moments/7(h_ground)
  Moments_sign/1 -> Aero Forces and Moments/8(Moments_sign)
  Propeller Torque/1 -> Display2/1, Abs1/1
  T_FaFb/1 -> M prop @Fb/1, F prop @ Fb/1
  Aero Forces and Moments/1(F_p) -> Display1/1, F prop @ Fb/2
  F prop @ Fb/1 -> M_PAF/2, Forces_prop @Fb/1
  r_p/1 -> M_PAF/1
  M_PAF/1 -> Display/1, Add/1
  M prop @Fb/1 -> Add/2
  Abs1/1 -> Prop_Torque_out/1
  Matrix  1-Norm1/1 -> Vx dimless/1
  mu/1 -> Coefficients/2(mu)
  Coefficients/4(C_Q) -> Aero Forces and Moments/4(C_Q)

== system Trim_Model/3 Copter Complete/Arms Dynamics: Forces and Moments/Arm 1 Dynamics/Arms Kinematics ==
  note: Input angles in rads
      |
      | 1. eta_1 (rad)  (Pan arm 1)
      | 2. gamma_1 (rad)  (Tirl arm 1)
  Angles (rad) : Inport
  Angles_dot (rad/s) : Inport  Port=2
  Add : Sum
  Add3 : Sum
  Bus Creator : BusCreator  Inputs=2
  Cross Product : vrlib/Utilities/Cross Product
  DCM Arm 1 : MATLAB Function  TreatAsAtomicUnit=on
  Demux : Demux  Outputs=2
  Demux3 : Demux  Outputs=2
  Fa->Fb : Product  Multiplication=Matrix(*)
  Gain : Gain  Gain=[1;0;0]
  Gain1 : Gain  Gain=[0;1;0]
  Gain6 : Gain  Gain=[1;0;0]
  Gain7 : Gain  Gain=[0;0;-1]
  Matrix Multiply : Product  Multiplication=Matrix(*)
  Transpose : dspmtrx3/Transpose  Hermitian=off  overflowFlag=off
  h arm : Constant  Value=h
  length arm : Constant  Value=l
  r_p1 (m) : Outport
  r_p1_dot (m/s) : Outport  Port=2
  Arm DCMs : Outport  Port=3
  omega^1_Ab (rad/s) : Outport  Port=4
  wires:
  DCM Arm 1/1(T_Fb_FA) -> Transpose/1, Bus Creator/1  "T^1_Fb,FA"
  Bus Creator/1 -> Arm DCMs/1
  Transpose/1 -> [T1_F_aFb], Bus Creator/2  "T^1_F_a,Fb"
  Angles (rad)/1 -> Demux/1
  Demux/1 -> DCM Arm 1/1(eta_1)
  Demux/2 -> DCM Arm 1/2(gamma_1)
  Angles_dot (rad/s)/1 -> Demux3/1
  Demux3/2 -> Gain1/1  "gamma_dot_1"
  Demux3/1 -> Gain/1  "eta_dot_1"
  Gain1/1 -> Matrix Multiply/2
  [T1_F_aFb] -> Matrix Multiply/1
  Matrix Multiply/1 -> Add/2
  Gain/1 -> Add/1
  Add/1 -> Cross Product/1, omega^1_Ab (rad/s)/1  "omega^1_Ab"
  Add3/1 -> r_p1 (m)/1  "r_p1 (m)"
  length arm/1 -> Gain6/1
  h arm/1 -> Gain7/1
  Gain7/1 -> Fa->Fb/2
  [T1_F_aFb] -> Fa->Fb/1
  Gain6/1 -> Add3/1
  Fa->Fb/1 -> Cross Product/2, Add3/2
  Cross Product/1 -> r_p1_dot (m/s)/1

== system Trim_Model/3 Copter Complete/Arms Dynamics: Forces and Moments/Arm 1 Dynamics/ESC-MOTOR dynamics ==
  note: 1) Only subsystems can be added as variant choices at this level
      | 2) Blocks cannot be connected at this level as connectivity is
      | automatically determined at simulation, based on the active variant
  Throttle : Inport
  Omega : Inport  Port=2
  Initial Omega : Inport  Port=3
  Prop Torque : Inport  Port=4
  ESC+Motor Dynamcis COMPLETED : Subsystem  TreatAsAtomicUnit=on  VariantObject=Variant_completed
  ESC+Motor Dynamcis SYMPLIFIED : Subsystem  TreatAsAtomicUnit=on  VariantObject=Variant_simple
  Omega_out : Outport
  Omega_dot_out : Outport  Port=2

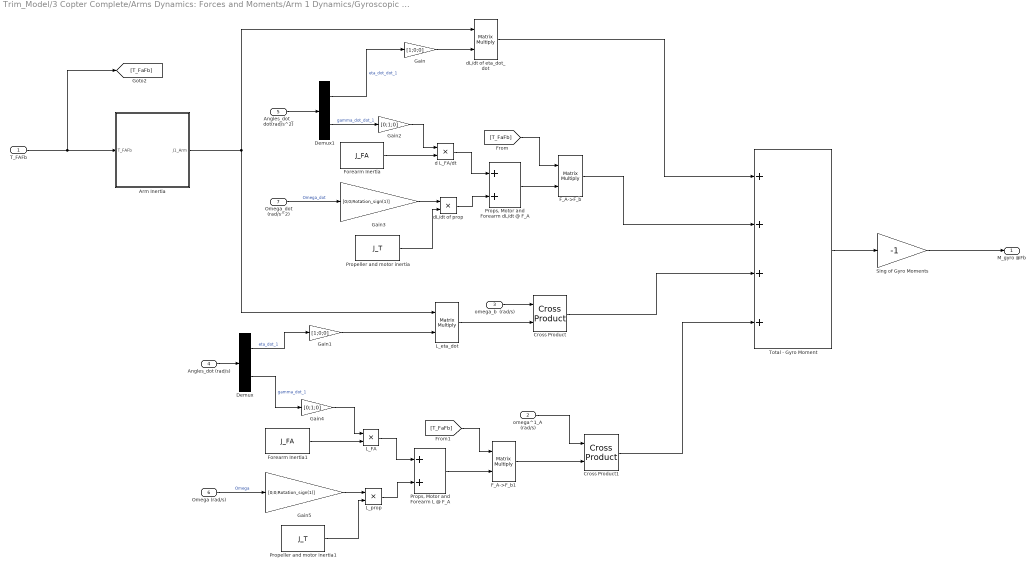
== system Trim_Model/3 Copter Complete/Arms Dynamics: Forces and Moments/Arm 1 Dynamics/Gyroscopic Moments ==
  T_FAFb : Inport
  omega^1_A  (rad/s) : Inport  Port=2
  omega_b  (rad/s) : Inport  Port=3
  Angles_dot (rad/s) : Inport  Port=4
  Angles_dot _dot(rad/s^2) : Inport  Port=5
  Omega (rad/s) : Inport  Port=6
  Omega_dot (rad/s^2) : Inport  Port=7
  Arm Inertia : MATLAB Function  TreatAsAtomicUnit=on
  Cross Product : vrlib/Utilities/Cross Product
  Cross Product1 : vrlib/Utilities/Cross Product
  Demux : Demux  Outputs=2
  Demux1 : Demux  Outputs=2
  F_A->F_b : Product  Multiplication=Matrix(*)
  F_A->F_b1 : Product  Multiplication=Matrix(*)
  Forearm Inertia : Constant  Value=J_FA
  Forearm Inertia1 : Constant  Value=J_FA
  Gain : Gain  Gain=[1;0;0]
  Gain1 : Gain  Gain=[1;0;0]
  Gain2 : Gain  Gain=[0;1;0]
  Gain3 : Gain  Gain=[0;0;Rotation_sign(1)]
  Gain4 : Gain  Gain=[0;1;0]
  Gain5 : Gain  Gain=[0;0;Rotation_sign(1)]
  L_FA : Product  Inputs=**
  L_eta_dot : Product  Multiplication=Matrix(*)
  L_prop : Product  Inputs=**
  Propeller and motor inertia : Constant  Value=J_T
  Propeller and motor inertia1 : Constant  Value=J_T
  "Props, Motor and Forearm L @ F_A" : Sum
  "Props, Motor and Forearm dL/dt @ F_A" : Sum
  Sing of Gyro Moments : Gain  Gain=-1
  Total - Gyro Moment : Sum  Inputs=++++
  d L_FA/dt : Product  Inputs=**
  dL/dt of eta_dot_dot : Product  Multiplication=Matrix(*)
  dL/dt of prop : Product  Inputs=**
  M_gyro @Fb : Outport
  wires:
  T_FAFb/1 -> [T_FaFb], Arm Inertia/1(T_FAFb)
  Angles_dot (rad/s)/1 -> Demux/1
  Angles_dot _dot(rad/s^2)/1 -> Demux1/1
  Demux1/1 -> Gain/1  "eta_dot_dot_1"
  Arm Inertia/1(J1_Arm) -> dL/dt of eta_dot_dot/1, L_eta_dot/1
  Gain/1 -> dL/dt of eta_dot_dot/2
  Gain1/1 -> L_eta_dot/2
  Demux/1 -> Gain1/1  "eta_dot_1"
  L_eta_dot/1 -> Cross Product/2
  omega_b  (rad/s)/1 -> Cross Product/1
  Demux1/2 -> Gain2/1  "gamma_dot_dot_1"
  Gain2/1 -> d L_FA/dt/1
  Forearm Inertia/1 -> d L_FA/dt/2
  Omega_dot (rad/s^2)/1 -> Gain3/1  "Omega_dot"
  Gain3/1 -> dL/dt of prop/1
  Propeller and motor inertia/1 -> dL/dt of prop/2
  d L_FA/dt/1 -> "Props, Motor and Forearm dL/dt @ F_A"/1
  dL/dt of prop/1 -> "Props, Motor and Forearm dL/dt @ F_A"/2
  Demux/2 -> Gain4/1  "gamma_dot_1"
  Gain4/1 -> L_FA/1
  Forearm Inertia1/1 -> L_FA/2
  Gain5/1 -> L_prop/1
  Propeller and motor inertia1/1 -> L_prop/2
  L_FA/1 -> "Props, Motor and Forearm L @ F_A"/1
  L_prop/1 -> "Props, Motor and Forearm L @ F_A"/2
  Omega (rad/s)/1 -> Gain5/1  "Omega"
  "Props, Motor and Forearm dL/dt @ F_A"/1 -> F_A->F_b/2
  F_A->F_b/1 -> Total - Gyro Moment/2
  dL/dt of eta_dot_dot/1 -> Total - Gyro Moment/1
  Cross Product/1 -> Total - Gyro Moment/3
  "Props, Motor and Forearm L @ F_A"/1 -> F_A->F_b1/2
  [T_FaFb] -> F_A->F_b/1
  [T_FaFb] -> F_A->F_b1/1
  F_A->F_b1/1 -> Cross Product1/2
  omega^1_A  (rad/s)/1 -> Cross Product1/1
  Cross Product1/1 -> Total - Gyro Moment/4
  Total - Gyro Moment/1 -> Sing of Gyro Moments/1
  Sing of Gyro Moments/1 -> M_gyro @Fb/1

== system Trim_Model/3 Copter Complete/Arms Dynamics: Forces and Moments/Arm 1 Dynamics/Servos Dynamics ==
  Com Angles (rad) : Inport
  Torques? : Inport  Port=2
  Demux : Demux  Outputs=2
  Derivative{,1..3} (4 alike) : Derivative  Commented=on  CoefficientInTFapproximation=0
  Mux : Mux  Inputs=2
  Mux1 : Mux  Commented=on  Inputs=2
  Mux2 : Mux  Commented=on  Inputs=2
  eta_1 : TransferFcn  Numerator=[1230]  Denominator=[1 50 1230]
  gamma_1 : TransferFcn  Numerator=[1230]  Denominator=[1 50 1230]
  Angles Arms (rad) : Outport
  Angles_dot (rad/s) : Outport  Port=2
  Angles_dot_dot (rad/s^2) : Outport  Port=3
  wires:
  Com Angles (rad)/1 -> Angles Arms (rad)/1, Demux/1
  Demux/1 -> eta_1/1
  Demux/2 -> gamma_1/1
  eta_1/1 -> Derivative/1, Mux/1
  gamma_1/1 -> Mux/2, Derivative1/1
  Mux1/1 -> Angles_dot (rad/s)/1
  Mux2/1 -> Angles_dot_dot (rad/s^2)/1
  Derivative1/1 -> Derivative3/1, Mux1/2
  Derivative2/1 -> Mux2/1
  Derivative3/1 -> Mux2/2
  Derivative/1 -> Mux1/1, Derivative2/1

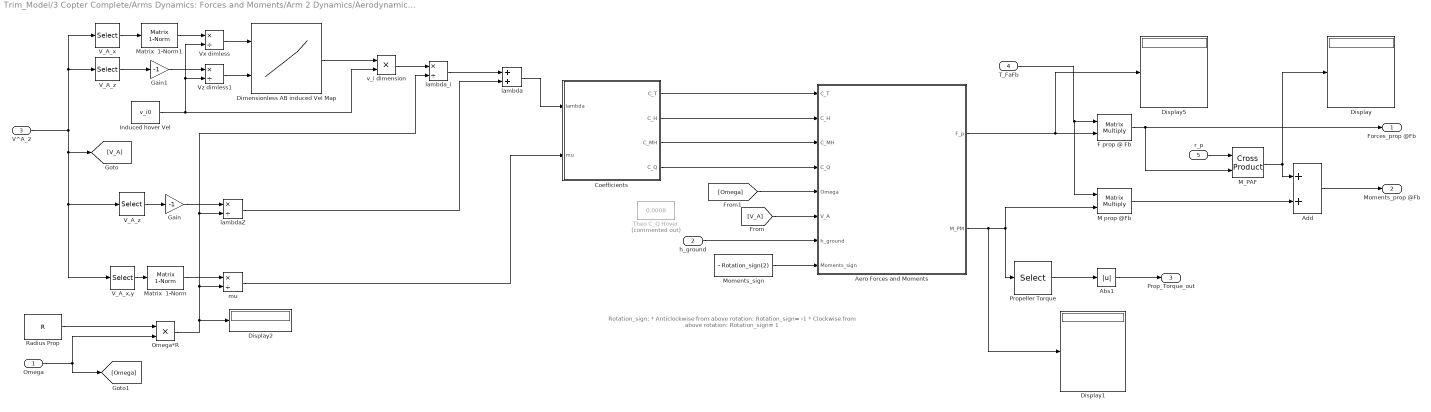
== system Trim_Model/3 Copter Complete/Arms Dynamics: Forces and Moments/Arm 2 Dynamics/Aerodynamics Propeller ==
  note: Rotation_sign:
      |
      | * Anticlockwise from above rotation: Rotation_sign= -1
      | * Clockwise from above rotation: Rotation_sign= 1
  Omega : Inport
  h_ground : Inport  Port=2
  V^A_2 : Inport  Port=3
  T_FaFb : Inport  Port=4
  r_p : Inport  Port=5
  Abs1 : Abs
  Add : Sum
  Aero Forces and Moments : MATLAB Function  TreatAsAtomicUnit=on
  Coefficients : MATLAB Function  TreatAsAtomicUnit=on
  Dimensionless AB induced Vel Map : Lookup_n-D  BreakpointsForDimension1=Vx_adim  BreakpointsForDimension2=Vz_adim  BreakpointsForDimension3=[5, 7]  Table=v_i_adim  ExtrapMethod=Clip  RndMeth=Simplest  InputSameDT=on
  Display{,1..2,5} (4 alike) : Display
  F prop @ Fb : Product  Multiplication=Matrix(*)
  Gain : Gain  Gain=-1
  Gain1 : Gain  Gain=-1
  Induced hover Vel : Constant  Value=v_i0
  M prop @Fb : Product  Multiplication=Matrix(*)
  M_PAF : vrlib/Utilities/Cross Product
  Matrix  1-Norm : dspmtrx3/Matrix  1-Norm  outputDataTypeStr=Inherit: Same as accumulator  outputLastDataTypeStr=Inherit: Same as accumulator  outputMin=[]  outputMax=[]  roundingMode=Floor  overflowMode=off
  Matrix  1-Norm1 : dspmtrx3/Matrix  1-Norm  outputDataTypeStr=Inherit: Same as accumulator  outputLastDataTypeStr=Inherit: Same as accumulator  outputMin=[]  outputMax=[]  roundingMode=Floor  overflowMode=off
  Moments_sign : Constant  Value=- Rotation_sign(2)
  Omega*R : Product  Inputs=**
  Propeller Torque : Selector  InputPortWidth=3  IndexOptions=Index vector (dialog)  Indices=3  OutputSizes=1
  Radius Prop : Constant  Value=R
  Theo C_Q Hover : Constant  Commented=on  Value=0.0008
  V_A_x : Selector  InputPortWidth=3  IndexOptions=Index vector (dialog)  Indices=[1 2]  OutputSizes=1
  V_A_x,y : Selector  InputPortWidth=3  IndexOptions=Index vector (dialog)  Indices=[1 2]  OutputSizes=1
  V_A_z : Selector  InputPortWidth=3  IndexOptions=Index vector (dialog)  Indices=3  OutputSizes=1
  "V_A_z " : Selector  InputPortWidth=3  IndexOptions=Index vector (dialog)  Indices=[3]  OutputSizes=1
  Vx dimless : Product  Inputs=*/
  Vz dimless1 : Product  Inputs=*/
  lambda : Sum
  lambdaZ : Product  Inputs=*/
  lambda_i : Product  Inputs=*/
  mu : Product  Inputs=*/
  v_i dimension : Product  Inputs=**
  Forces_prop @Fb : Outport
  Moments_prop @Fb : Outport  Port=2
  Prop_Torque_out : Outport  Port=3
  wires:
  Abs1/1 -> Prop_Torque_out/1
  M prop @Fb/1 -> Add/2
  M_PAF/1 -> Add/1, Display/1
  r_p/1 -> M_PAF/1
  F prop @ Fb/1 -> Forces_prop @Fb/1, M_PAF/2
  Aero Forces and Moments/1(F_p) -> Display5/1, F prop @ Fb/2
  T_FaFb/1 -> F prop @ Fb/1, M prop @Fb/1
  Propeller Torque/1 -> Abs1/1
  Moments_sign/1 -> Aero Forces and Moments/8(Moments_sign)
  h_ground/1 -> Aero Forces and Moments/7(h_ground)
  Add/1 -> Moments_prop @Fb/1
  Aero Forces and Moments/2(M_PM) -> Display1/1, M prop @Fb/2, Propeller Torque/1
  [Omega] -> Aero Forces and Moments/5(Omega)
  [V_A] -> Aero Forces and Moments/6(V_A)
  Coefficients/4(C_Q) -> Aero Forces and Moments/4(C_Q)
  Coefficients/3(C_MH) -> Aero Forces and Moments/3(C_MH)
  Coefficients/2(C_H) -> Aero Forces and Moments/2(C_H)
  Coefficients/1(C_T) -> Aero Forces and Moments/1(C_T)
  mu/1 -> Coefficients/2(mu)
  lambda/1 -> Coefficients/1(lambda)
  lambdaZ/1 -> lambda/2
  lambda_i/1 -> lambda/1
  Gain/1 -> lambdaZ/1
  "V_A_z "/1 -> Gain/1
  v_i dimension/1 -> lambda_i/1
  Dimensionless AB induced Vel Map/1 -> v_i dimension/1
  Vz dimless1/1 -> Dimensionless AB induced Vel Map/2
  Vx dimless/1 -> Dimensionless AB induced Vel Map/1
  Omega*R/1 -> Display2/1, lambda_i/2, lambdaZ/2, mu/2
  Matrix  1-Norm/1 -> mu/1
  V_A_x,y/1 -> Matrix  1-Norm/1
  Omega/1 -> [Omega], Omega*R/2
  Radius Prop/1 -> Omega*R/1
  V^A_2/1 -> V_A_z/1, V_A_x/1, V_A_x,y/1, "V_A_z "/1, [V_A]
  V_A_x/1 -> Matrix  1-Norm1/1
  V_A_z/1 -> Gain1/1
  Induced hover Vel/1 -> Vz dimless1/2, Vx dimless/2, v_i dimension/2
  Gain1/1 -> Vz dimless1/1
  Matrix  1-Norm1/1 -> Vx dimless/1

== system Trim_Model/3 Copter Complete/Arms Dynamics: Forces and Moments/Arm 2 Dynamics/Arms Kinematics ==
  note: Input angles in rads
      |
      | 1. eta_2 (rad)  (Pan arm 2)
      | 2. gamma_2 (rad)  (Tilt arm 2)
  Angles (rad) : Inport
  Angles_dot (rad/s) : Inport  Port=2
  Add : Sum
  Add3 : Sum
  Bus Creator : BusCreator  Inputs=2
  Cross Product : vrlib/Utilities/Cross Product
  DCM Arm 2 : MATLAB Function  TreatAsAtomicUnit=on
  Demux : Demux  Outputs=2
  Demux3 : Demux  Outputs=2
  Fa->Fb : Product  Multiplication=Matrix(*)
  Gain6 : Gain  Gain=[0;1;0]
  Gain7 : Gain  Gain=[0;0;-1]
  Gain8 : Gain  Gain=[-1/2;sqrt(3)/2;0]
  Gain9 : Gain  Gain=[1;0;0]
  Matrix Multiply : Product  Multiplication=Matrix(*)
  Transpose : dspmtrx3/Transpose  Hermitian=off  overflowFlag=off
  h arm : Constant  Value=h
  length arm : Constant  Value=l
  r_p2 (m) : Outport
  r_p2_dot (m/s) : Outport  Port=2
  Arm DCMs : Outport  Port=3
  omega^2_Ab (rad/s) : Outport  Port=4
  wires:
  Cross Product/1 -> r_p2_dot (m/s)/1
  Fa->Fb/1 -> Add3/2, Cross Product/2
  Gain8/1 -> Add3/1
  [T2_F_aFb] -> Fa->Fb/1
  Gain7/1 -> Fa->Fb/2
  h arm/1 -> Gain7/1
  length arm/1 -> Gain8/1
  Add3/1 -> r_p2 (m)/1  "r_p2 (m)"
  Add/1 -> omega^2_Ab (rad/s)/1, Cross Product/1  "omega^2_Ab"
  Gain6/1 -> Add/1
  Matrix Multiply/1 -> Add/2
  [T2_F_aFb] -> Matrix Multiply/1
  Gain9/1 -> Matrix Multiply/2
  Demux3/1 -> Gain6/1  "eta_dot_2"
  Demux3/2 -> Gain9/1  "gamma_dot_2"
  Angles_dot (rad/s)/1 -> Demux3/1
  Demux/2 -> DCM Arm 2/2(gamma_2)
  Demux/1 -> DCM Arm 2/1(eta_2)
  Angles (rad)/1 -> Demux/1
  Transpose/1 -> Bus Creator/2, [T2_F_aFb]  "T^2_F_a,Fb"
  Bus Creator/1 -> Arm DCMs/1
  DCM Arm 2/1(T_Fb_FA) -> Bus Creator/1, Transpose/1  "T^2_Fb,FA"

== system Trim_Model/3 Copter Complete/Arms Dynamics: Forces and Moments/Arm 2 Dynamics/ESC-MOTOR dynamics1 ==
  note: 1) Only subsystems can be added as variant choices at this level
      | 2) Blocks cannot be connected at this level as connectivity is
      | automatically determined at simulation, based on the active variant
  Throttle : Inport
  Omega : Inport  Port=2
  Initial Omega : Inport  Port=3
  Prop Torque : Inport  Port=4
  ESC+Motor Dynamcis COMPLETED : Subsystem  TreatAsAtomicUnit=on  VariantObject=Variant_completed
  ESC+Motor Dynamcis SYMPLIFIED : Subsystem  TreatAsAtomicUnit=on  VariantObject=Variant_simple
  Omega_out : Outport
  Omega_dot_out : Outport  Port=2

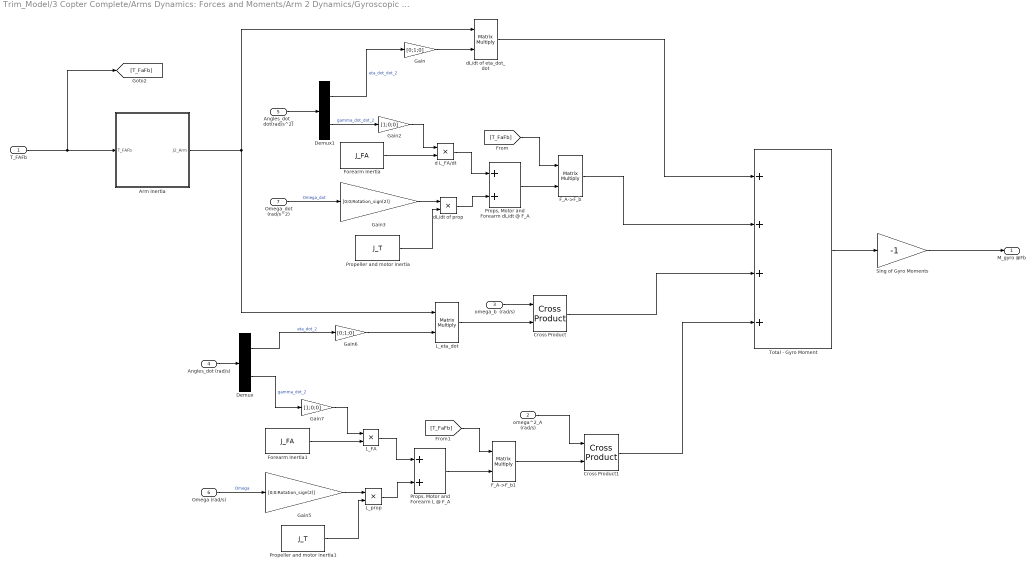
== system Trim_Model/3 Copter Complete/Arms Dynamics: Forces and Moments/Arm 2 Dynamics/Gyroscopic Moments ==
  T_FAFb : Inport
  omega^2_A  (rad/s) : Inport  Port=2
  omega_b  (rad/s) : Inport  Port=3
  Angles_dot (rad/s) : Inport  Port=4
  Angles_dot _dot(rad/s^2) : Inport  Port=5
  Omega (rad/s) : Inport  Port=6
  Omega_dot (rad/s^2) : Inport  Port=7
  Arm Inertia : MATLAB Function  TreatAsAtomicUnit=on
  Cross Product : vrlib/Utilities/Cross Product
  Cross Product1 : vrlib/Utilities/Cross Product
  Demux : Demux  Outputs=2
  Demux1 : Demux  Outputs=2
  F_A->F_b : Product  Multiplication=Matrix(*)
  F_A->F_b1 : Product  Multiplication=Matrix(*)
  Forearm Inertia : Constant  Value=J_FA
  Forearm Inertia1 : Constant  Value=J_FA
  Gain : Gain  Gain=[0;1;0]
  Gain2 : Gain  Gain=[1;0;0]
  Gain3 : Gain  Gain=[0;0;Rotation_sign(2)]
  Gain5 : Gain  Gain=[0;0;Rotation_sign(2)]
  Gain6 : Gain  Gain=[0;1;0]
  Gain7 : Gain  Gain=[1;0;0]
  L_FA : Product  Inputs=**
  L_eta_dot : Product  Multiplication=Matrix(*)
  L_prop : Product  Inputs=**
  Propeller and motor inertia : Constant  Value=J_T
  Propeller and motor inertia1 : Constant  Value=J_T
  "Props, Motor and Forearm L @ F_A" : Sum
  "Props, Motor and Forearm dL/dt @ F_A" : Sum
  Sing of Gyro Moments : Gain  Gain=-1
  Total - Gyro Moment : Sum  Inputs=++++
  d L_FA/dt : Product  Inputs=**
  dL/dt of eta_dot_dot : Product  Multiplication=Matrix(*)
  dL/dt of prop : Product  Inputs=**
  M_gyro @Fb : Outport
  wires:
  Sing of Gyro Moments/1 -> M_gyro @Fb/1
  Total - Gyro Moment/1 -> Sing of Gyro Moments/1
  Cross Product1/1 -> Total - Gyro Moment/4
  omega^2_A  (rad/s)/1 -> Cross Product1/1
  F_A->F_b1/1 -> Cross Product1/2
  [T_FaFb] -> F_A->F_b1/1
  [T_FaFb] -> F_A->F_b/1
  "Props, Motor and Forearm L @ F_A"/1 -> F_A->F_b1/2
  Cross Product/1 -> Total - Gyro Moment/3
  dL/dt of eta_dot_dot/1 -> Total - Gyro Moment/1
  F_A->F_b/1 -> Total - Gyro Moment/2
  "Props, Motor and Forearm dL/dt @ F_A"/1 -> F_A->F_b/2
  Omega (rad/s)/1 -> Gain5/1  "Omega"
  L_prop/1 -> "Props, Motor and Forearm L @ F_A"/2
  L_FA/1 -> "Props, Motor and Forearm L @ F_A"/1
  Propeller and motor inertia1/1 -> L_prop/2
  Gain5/1 -> L_prop/1
  Forearm Inertia1/1 -> L_FA/2
  Gain7/1 -> L_FA/1
  Demux/2 -> Gain7/1  "gamma_dot_2"
  dL/dt of prop/1 -> "Props, Motor and Forearm dL/dt @ F_A"/2
  d L_FA/dt/1 -> "Props, Motor and Forearm dL/dt @ F_A"/1
  Propeller and motor inertia/1 -> dL/dt of prop/2
  Gain3/1 -> dL/dt of prop/1
  Omega_dot (rad/s^2)/1 -> Gain3/1  "Omega_dot"
  Forearm Inertia/1 -> d L_FA/dt/2
  Gain2/1 -> d L_FA/dt/1
  Demux1/2 -> Gain2/1  "gamma_dot_dot_2"
  omega_b  (rad/s)/1 -> Cross Product/1
  L_eta_dot/1 -> Cross Product/2
  Demux/1 -> Gain6/1  "eta_dot_2"
  Gain6/1 -> L_eta_dot/2
  Gain/1 -> dL/dt of eta_dot_dot/2
  Arm Inertia/1(J2_Arm) -> L_eta_dot/1, dL/dt of eta_dot_dot/1
  Demux1/1 -> Gain/1  "eta_dot_dot_2"
  Angles_dot _dot(rad/s^2)/1 -> Demux1/1
  Angles_dot (rad/s)/1 -> Demux/1
  T_FAFb/1 -> Arm Inertia/1(T_FAFb), [T_FaFb]

== system Trim_Model/3 Copter Complete/Arms Dynamics: Forces and Moments/Arm 2 Dynamics/Servos Dynamics ==
  Com Angles (rad) : Inport
  Torques? : Inport  Port=2
  Demux : Demux  Outputs=2
  Derivative : Derivative  CoefficientInTFapproximation=0
  Derivative1 : Derivative  Commented=on  CoefficientInTFapproximation=0
  Derivative2 : Derivative  Commented=on  CoefficientInTFapproximation=0
  Derivative3 : Derivative  Commented=on  CoefficientInTFapproximation=0
  Mux : Mux  Inputs=2
  Mux1 : Mux  Commented=on  Inputs=2
  Mux2 : Mux  Commented=on  Inputs=2
  eta_2 : TransferFcn  Numerator=[1230]  Denominator=[1 50 1230]
  gamma_2 : TransferFcn  Numerator=[1230]  Denominator=[1 50 1230]
  Angles Arms (rad) : Outport
  Angles_dot (rad/s) : Outport  Port=2
  Angles_dot_dot (rad/s^2) : Outport  Port=3
  wires:
  Derivative/1 -> Derivative2/1, Mux1/1
  Derivative3/1 -> Mux2/2
  Derivative2/1 -> Mux2/1
  Derivative1/1 -> Mux1/2, Derivative3/1
  Mux2/1 -> Angles_dot_dot (rad/s^2)/1
  Mux1/1 -> Angles_dot (rad/s)/1
  gamma_2/1 -> Derivative1/1, Mux/2
  eta_2/1 -> Mux/1, Derivative/1
  Com Angles (rad)/1 -> Angles Arms (rad)/1, Demux/1
  Demux/2 -> gamma_2/1
  Demux/1 -> eta_2/1
